simulink model "LC_Oscilation"  (R2016b)
settings: Solver=VariableStepAuto  StartTime=0.0  StopTime=10.0  RelTol=1e-3
libraries: simrfV2elements x3, simrfV2sources1 x2
settings Model: Creator=Dhiman Sarkar  LastModifiedBy=Dhiman Sarkar

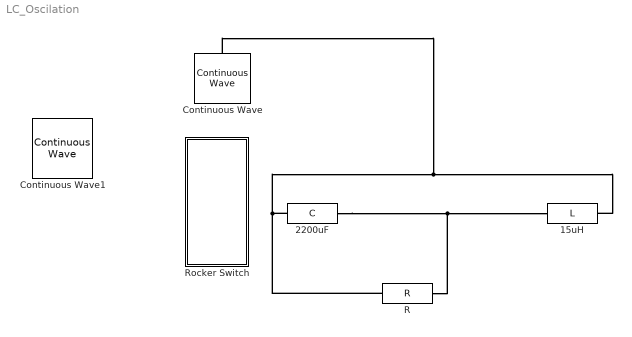
== system LC_Oscilation ==
  15uH : simrfV2elements/L  classname=inductor  Inductance=150 uH
  2200uF : simrfV2elements/C  classname=capacitor  Capacitance=2200 uF
  Continuous Wave : simrfV2sources1/Continuous Wave  CWSourceType=Ideal voltage  Z0=0  IVoltage=0 V  ICurrent=0 A  MagPower=0 W  QVoltage=0 V  QCurrent=0 A  AnglePower=0  CarrierFreq=0 Hz  InternalGrounding=on
  Continuous Wave1 : simrfV2sources1/Continuous Wave  CWSourceType=Ideal voltage  Z0=0  IVoltage=0 V  ICurrent=0 A  MagPower=0 W  QVoltage=0 V  QCurrent=0 A  AnglePower=0  CarrierFreq=0 Hz  InternalGrounding=on
  R : simrfV2elements/R  classname=resistor  Resistance=50 Ohm  AddNoise=on
  Rocker Switch : Subsystem  DialogController=hmiCreateDDGDialog  IsWebBlock=on  mask(MWDashboardBlock){webBlockId=ecb7d6dc-4746-4033-a3bf-375ba57c283b, webBlockType=rockerswitch, ShowInLibBrowser=on, ShowInitialText=on, HMISrcModelName=LC_Oscilation}
      mask prompts: webBlockId "WebBlock Id"; webBlockType "WebBlock Type"; HMISrcModelName "Source Model"
      mask help: SimulinkHMI:dialogs:SwitchDialogDesc
      mask Help: helpview([docroot '/mapfiles/simulink.map'], 'hmi_rocker_switch')
      mask Display:
      | if strcmp(get_param(bdroot(gcb),'BlockDiagramType'), 'library')
      |     image([(matlabroot) '/toolbox/simulink/hmi/icons/RockerSwitch.png']);
      | end
  connections:
  2200uF/RConn1 -- R/RConn1 -- 15uH/LConn1
  2200uF/LConn1 -- Continuous Wave/LConn1 -- 15uH/RConn1 -- R/LConn1

== system LC_Oscilation/Rocker Switch ==
